simulink model "3DoFManipulatorWithBLDCM_SIMULATION"  (R2023b)
settings: Solver=VariableStepAuto  StartTime=0.0  StopTime=10  MaxStep=1e-4  RelTol=1e-3
undefined symbols (not defined in the file): X, Y, Z
libraries: spsMosfetLib x18, sm_lib x11, nesl_utility x7, eeGeneralControl x6, spsDCVoltageSourceLib x3, spsGroundLib x3, spsThreePhaseSeriesRLCBranchLib x3, spsThreePhaseVIMeasurementLib x3, slpidlib x3, sps_lib x1
(part 2 of 3)

== system 3DoFManipulatorWithBLDCM_SIMULATION/Feedforward Control/PWM LINK1 ==
  target position : Inport
  target velocity : Inport  Port=2
  actual position : Inport  Port=3
  CCW : Scope
  Duty Cycle : Scope
  MOTOR_SPEED_BLOCK3 : MATLAB Function  TreatAsAtomicUnit=on
  Mux : Mux  Inputs=2
  PID Controller Position : slpidlib/PID Controller  Controller=PID  Form=Parallel  TimeDomain=Continuous-time  UseExternalTs=off  SampleTime=-1  IntegratorMethod=Forward Euler  FilterMethod=Forward Euler  ControllerParametersSource=internal  P=800  I=20000  UseKiTs=off  D=0  N=100  UseFilter=on  TunerSelectOption=Transfer Function Based (PID Tuner App)  InitialConditionSource=internal  InitialConditionForIntegrator=0  InitialConditionForFilter=0  DifferentiatorICPrevScaledInput=0  ExternalReset=none  TrackingMode=off  Kt=1  LimitOutput=off  SatLimitsSource=internal  UpperSaturationLimit=inf  LowerSaturationLimit=-inf  LinearizeAsGain=on  AntiWindupMode=none  Kb=1  LimitIntegrator=off  UpperIntegratorSaturationLimit=inf  LowerIntegratorSaturationLimit=-inf  POutMin=[]  POutMax=[]  IOutMin=[]  IOutMax=[]  DOutMin=[]  DOutMax=[]  NOutMin=[]  NOutMax=[]  SumOutMin=[]  SumOutMax=[]  SaturationOutMin=[]  SaturationOutMax=[]  PParamMin=[]  PParamMax=[]  IParamMin=[]  IParamMax=[]  DParamMin=[]  DParamMax=[]  NParamMin=[]  NParamMax=[]  KbParamMin=[]  KbParamMax=[]  KtParamMin=[]  KtParamMax=[]  KbOutMin=[]  KbOutMax=[]  KtOutMin=[]  KtOutMax=[]  IntegratorOutMin=[]  IntegratorOutMax=[]  FilterOutMin=[]  FilterOutMax=[]  SumI1OutMin=[]  SumI1OutMax=[]  SumI2OutMin=[]  SumI2OutMax=[]  SumI3OutMin=[]  SumI3OutMax=[]  SumI4OutMin=[]  SumI4OutMax=[]  SumDOutMin=[]  SumDOutMax=[]  DifferentiatorOutMin=[]  DifferentiatorOutMax=[]  FilterDiffOutCoefMin=[]  FilterDiffOutCoefMax=[]  ReciprocalOutMin=[]  ReciprocalOutMax=[]  SumDenOutMin=[]  SumDenOutMax=[]  SumNumOutMin=[]  SumNumOutMax=[]  DivideOutMin=[]  DivideOutMax=[]  UdiffTsProdOutMin=[]  UdiffTsProdOutMax=[]  NTsProdOutMin=[]  NTsProdOutMax=[]  UintegralTsProdOutMin=[]  UintegralTsProdOutMax=[]  UngainTsProdOutMin=[]  UngainTsProdOutMax=[]  ClampingZeroOutDataTypeStr=Inherit: Inherit via back propagation  ClampingZeroOutMin=[]  ClampingZeroOutMax=[]  FilterDenConstantOutDataTypeStr=Inherit: Inherit via back propagation  FilterDenConstantOutMin=[]  FilterDenConstantOutMax=[]  PCopyOutDataTypeStr=Inherit: Inherit via back propagation  PCopyOutMin=[]  PCopyOutMax=[]  NCopyOutDataTypeStr=Inherit: Inherit via back propagation  NCopyOutMin=[]  NCopyOutMax=[]  IntegratorContinuousStateAttributes=''  IntegratorStateMustResolveToSignalObject=off  IntegratorRTWStateStorageClass=Auto  FilterContinuousStateAttributes=''  FilterStateMustResolveToSignalObject=off  FilterRTWStateStorageClass=Auto  ParallelPVariant=InternalParameters  IdealPVariant=Disabled  IVariant=InternalParameters  DVariant=InternalParameters  IntegratorVariant=Continuous  SatVariant=Disabled  AWVariant=Passthrough  PCopyVariant=Disabled  TRVariant=Disabled  FdbkBlocksVariant=Forward  IdealPFdbkVariant=Disabled  SatFdbkVariant=Disabled  DerivativeFilterVariant=ContFilter  NVariant=InternalParameters  NCopyVariant=Disabled  FilterICVariant=InternalICsFilter  IntegratorICVariant=InternalICs  ExternalResetVariant=Disabled  TRSumVariant=Passthrough  SumFdbkVariant=Disabled  SumVariant=Sum_PID  TsampFilterVariant=InternalTs  TsampNgainVariant=Passthrough  TsampIntegralVariant=Disabled_SignalSpec  ExternalSaturationOutDataTypeStr=Inherit: Same as second input
  PWM-Signal : Scope
  Variable Pulse Generator : VariablePulseGenerator  AllowZeroPulseWidth=on  SampleTime=0.1
  diff_pos : MATLAB Function  TreatAsAtomicUnit=on  SystemSampleTime=1e-4
  PWM_L1 : Outport
  wires:
  diff_pos/2(CCW) -> CCW/1, [CCW]
  diff_pos/1(diff_pos) -> PID Controller Position/1
  Mux/1 -> PWM_L1/1
  PID Controller Position/1 -> MOTOR_SPEED_BLOCK3/1(e_diff)
  Variable Pulse Generator/1 -> Mux/2, PWM-Signal/1
  MOTOR_SPEED_BLOCK3/2(p) -> Variable Pulse Generator/2
  [CCW] -> Mux/1
  MOTOR_SPEED_BLOCK3/1(dC) -> Duty Cycle/1, Variable Pulse Generator/1
  target position/1 -> diff_pos/1(t_pos)
  actual position/1 -> diff_pos/3(a_pos)
  target velocity/1 -> diff_pos/2(t_vel)

== system 3DoFManipulatorWithBLDCM_SIMULATION/Feedforward Control/PWM LINK2 ==
  target position : Inport
  target velocity : Inport  Port=2
  actual position : Inport  Port=3
  CCW : Scope
  Duty Cycle : Scope
  MOTOR_SPEED_BLOCK3 : MATLAB Function  TreatAsAtomicUnit=on
  Mux : Mux  Inputs=2
  PID Controller Position : slpidlib/PID Controller  Controller=PID  Form=Parallel  TimeDomain=Continuous-time  UseExternalTs=off  SampleTime=-1  IntegratorMethod=Forward Euler  FilterMethod=Forward Euler  ControllerParametersSource=internal  P=2000  I=20000  UseKiTs=off  D=0  N=100  UseFilter=on  TunerSelectOption=Transfer Function Based (PID Tuner App)  InitialConditionSource=internal  InitialConditionForIntegrator=0  InitialConditionForFilter=0  DifferentiatorICPrevScaledInput=0  ExternalReset=none  TrackingMode=off  Kt=1  LimitOutput=off  SatLimitsSource=internal  UpperSaturationLimit=inf  LowerSaturationLimit=-inf  LinearizeAsGain=on  AntiWindupMode=none  Kb=1  LimitIntegrator=off  UpperIntegratorSaturationLimit=inf  LowerIntegratorSaturationLimit=-inf  POutMin=[]  POutMax=[]  IOutMin=[]  IOutMax=[]  DOutMin=[]  DOutMax=[]  NOutMin=[]  NOutMax=[]  SumOutMin=[]  SumOutMax=[]  SaturationOutMin=[]  SaturationOutMax=[]  PParamMin=[]  PParamMax=[]  IParamMin=[]  IParamMax=[]  DParamMin=[]  DParamMax=[]  NParamMin=[]  NParamMax=[]  KbParamMin=[]  KbParamMax=[]  KtParamMin=[]  KtParamMax=[]  KbOutMin=[]  KbOutMax=[]  KtOutMin=[]  KtOutMax=[]  IntegratorOutMin=[]  IntegratorOutMax=[]  FilterOutMin=[]  FilterOutMax=[]  SumI1OutMin=[]  SumI1OutMax=[]  SumI2OutMin=[]  SumI2OutMax=[]  SumI3OutMin=[]  SumI3OutMax=[]  SumI4OutMin=[]  SumI4OutMax=[]  SumDOutMin=[]  SumDOutMax=[]  DifferentiatorOutMin=[]  DifferentiatorOutMax=[]  FilterDiffOutCoefMin=[]  FilterDiffOutCoefMax=[]  ReciprocalOutMin=[]  ReciprocalOutMax=[]  SumDenOutMin=[]  SumDenOutMax=[]  SumNumOutMin=[]  SumNumOutMax=[]  DivideOutMin=[]  DivideOutMax=[]  UdiffTsProdOutMin=[]  UdiffTsProdOutMax=[]  NTsProdOutMin=[]  NTsProdOutMax=[]  UintegralTsProdOutMin=[]  UintegralTsProdOutMax=[]  UngainTsProdOutMin=[]  UngainTsProdOutMax=[]  ClampingZeroOutDataTypeStr=Inherit: Inherit via back propagation  ClampingZeroOutMin=[]  ClampingZeroOutMax=[]  FilterDenConstantOutDataTypeStr=Inherit: Inherit via back propagation  FilterDenConstantOutMin=[]  FilterDenConstantOutMax=[]  PCopyOutDataTypeStr=Inherit: Inherit via back propagation  PCopyOutMin=[]  PCopyOutMax=[]  NCopyOutDataTypeStr=Inherit: Inherit via back propagation  NCopyOutMin=[]  NCopyOutMax=[]  IntegratorContinuousStateAttributes=''  IntegratorStateMustResolveToSignalObject=off  IntegratorRTWStateStorageClass=Auto  FilterContinuousStateAttributes=''  FilterStateMustResolveToSignalObject=off  FilterRTWStateStorageClass=Auto  ParallelPVariant=InternalParameters  IdealPVariant=Disabled  IVariant=InternalParameters  DVariant=InternalParameters  IntegratorVariant=Continuous  SatVariant=Disabled  AWVariant=Passthrough  PCopyVariant=Disabled  TRVariant=Disabled  FdbkBlocksVariant=Forward  IdealPFdbkVariant=Disabled  SatFdbkVariant=Disabled  DerivativeFilterVariant=ContFilter  NVariant=InternalParameters  NCopyVariant=Disabled  FilterICVariant=InternalICsFilter  IntegratorICVariant=InternalICs  ExternalResetVariant=Disabled  TRSumVariant=Passthrough  SumFdbkVariant=Disabled  SumVariant=Sum_PID  TsampFilterVariant=InternalTs  TsampNgainVariant=Passthrough  TsampIntegralVariant=Disabled_SignalSpec  ExternalSaturationOutDataTypeStr=Inherit: Same as second input
  PWM-Signal : Scope
  Variable Pulse Generator : VariablePulseGenerator  AllowZeroPulseWidth=on  SampleTime=0.1
  diff_pos : MATLAB Function  TreatAsAtomicUnit=on  SystemSampleTime=1e-4
  PWM_L2 : Outport
  wires:
  [CCW] -> Mux/1
  Variable Pulse Generator/1 -> Mux/2, PWM-Signal/1
  MOTOR_SPEED_BLOCK3/2(p) -> Variable Pulse Generator/2
  MOTOR_SPEED_BLOCK3/1(dC) -> Variable Pulse Generator/1, Duty Cycle/1
  Mux/1 -> PWM_L2/1
  PID Controller Position/1 -> MOTOR_SPEED_BLOCK3/1(e_diff)
  diff_pos/1(diff_pos) -> PID Controller Position/1
  diff_pos/2(CCW) -> CCW/1, [CCW]
  target position/1 -> diff_pos/1(t_pos)
  actual position/1 -> diff_pos/3(a_pos)
  target velocity/1 -> diff_pos/2(t_vel)

== system 3DoFManipulatorWithBLDCM_SIMULATION/Trajectorie Control/Subsystem ==
  From Workspace : FromWorkspace  VariableName=ts1_q0_pos
  From Workspace1 : FromWorkspace  VariableName=ts1_q1_pos
  From Workspace2 : FromWorkspace  VariableName=ts1_q2_pos
  From Workspace3 : FromWorkspace  VariableName=ts1_q0_vel
  From Workspace4 : FromWorkspace  VariableName=ts1_q1_vel
  From Workspace5 : FromWorkspace  VariableName=ts1_q2_vel
  From Workspace6 : FromWorkspace  VariableName=ts1_q0_acc
  From Workspace7 : FromWorkspace  VariableName=ts1_q1_acc
  From Workspace8 : FromWorkspace  VariableName=ts1_q2_acc
  Mux{,5..7} (4 alike) : Mux  Inputs=3
  Trajektorie 1 : Outport
  wires:
  From Workspace4/1 -> Mux6/2
  From Workspace3/1 -> Mux6/1
  From Workspace5/1 -> Mux6/3
  From Workspace6/1 -> Mux7/1
  From Workspace2/1 -> Mux5/3
  From Workspace8/1 -> Mux7/3
  From Workspace1/1 -> Mux5/2
  From Workspace/1 -> Mux5/1
  From Workspace7/1 -> Mux7/2
  Mux5/1 -> Mux/1
  Mux6/1 -> Mux/2
  Mux7/1 -> Mux/3
  Mux/1 -> Trajektorie 1/1

== system 3DoFManipulatorWithBLDCM_SIMULATION/Trajectorie Control/Subsystem1 ==
  From Workspace : FromWorkspace  VariableName=ts2_q0_pos
  From Workspace1 : FromWorkspace  VariableName=ts2_q1_pos
  From Workspace2 : FromWorkspace  VariableName=ts2_q2_pos
  From Workspace3 : FromWorkspace  VariableName=ts2_q0_vel
  From Workspace4 : FromWorkspace  VariableName=ts2_q1_vel
  From Workspace5 : FromWorkspace  VariableName=ts2_q2_vel
  From Workspace6 : FromWorkspace  VariableName=ts2_q0_acc
  From Workspace7 : FromWorkspace  VariableName=ts2_q1_acc
  From Workspace8 : FromWorkspace  VariableName=ts2_q2_acc
  Mux{,5..7} (4 alike) : Mux  Inputs=3
  Trajektorie 2 : Outport
  wires:
  From Workspace4/1 -> Mux6/2
  From Workspace3/1 -> Mux6/1
  From Workspace5/1 -> Mux6/3
  From Workspace6/1 -> Mux7/1
  From Workspace2/1 -> Mux5/3
  From Workspace8/1 -> Mux7/3
  From Workspace1/1 -> Mux5/2
  From Workspace/1 -> Mux5/1
  From Workspace7/1 -> Mux7/2
  Mux/1 -> Trajektorie 2/1
  Mux7/1 -> Mux/3
  Mux5/1 -> Mux/1
  Mux6/1 -> Mux/2

== system 3DoFManipulatorWithBLDCM_SIMULATION/Trajectorie Control/Subsystem2 ==
  From Workspace : FromWorkspace  VariableName=ts3_q0_pos
  From Workspace1 : FromWorkspace  VariableName=ts3_q1_pos
  From Workspace2 : FromWorkspace  VariableName=ts3_q2_pos
  From Workspace3 : FromWorkspace  VariableName=ts3_q0_vel
  From Workspace4 : FromWorkspace  VariableName=ts3_q1_vel
  From Workspace5 : FromWorkspace  VariableName=ts3_q2_vel
  From Workspace6 : FromWorkspace  VariableName=ts3_q0_acc
  From Workspace7 : FromWorkspace  VariableName=ts3_q1_acc
  From Workspace8 : FromWorkspace  VariableName=ts3_q2_acc
  Mux{,5..7} (4 alike) : Mux  Inputs=3
  Trajektorie 3 : Outport
  wires:
  From Workspace4/1 -> Mux6/2
  From Workspace3/1 -> Mux6/1
  From Workspace5/1 -> Mux6/3
  From Workspace6/1 -> Mux7/1
  From Workspace2/1 -> Mux5/3
  From Workspace8/1 -> Mux7/3
  From Workspace1/1 -> Mux5/2
  From Workspace/1 -> Mux5/1
  From Workspace7/1 -> Mux7/2
  Mux/1 -> Trajektorie 3/1
  Mux7/1 -> Mux/3
  Mux5/1 -> Mux/1
  Mux6/1 -> Mux/2

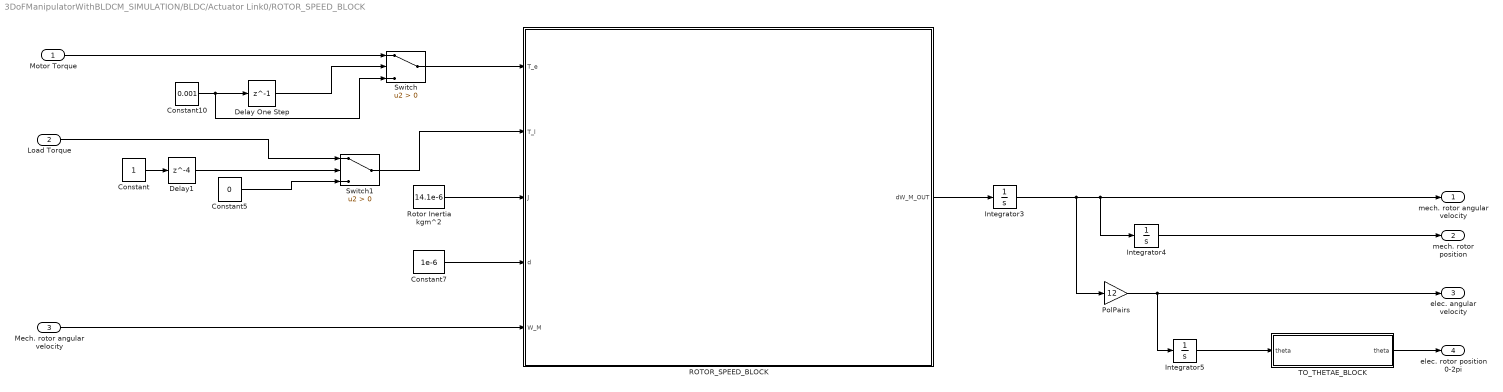
== system 3DoFManipulatorWithBLDCM_SIMULATION/BLDC/Actuator Link0/ROTOR_SPEED_BLOCK ==
  Motor Torque : Inport
  Load Torque : Inport  Port=2
  Mech. rotor angular velocity : Inport  Port=3
  Constant : Constant
  Constant10 : Constant  Value=0.001
  Constant5 : Constant  Value=0
  Constant7 : Constant  Value=1e-6
  Delay One Step : Delay  DelayLength=1
  Delay1 : Delay  DelayLength=4
  Integrator3 : Integrator
  Integrator4 : Integrator
  Integrator5 : Integrator
  PolPairs : Gain  Gain=12
  ROTOR_SPEED_BLOCK : MATLAB Function  TreatAsAtomicUnit=on
  Rotor Inertia kgm^2 : Constant  Value=14.1e-6
  Switch : Switch  Criteria=u2 > Threshold  SaturateOnIntegerOverflow=off  InputSameDT=off
  Switch1 : Switch  Criteria=u2 > Threshold  SaturateOnIntegerOverflow=off  InputSameDT=off
  TO_THETAE_BLOCK : MATLAB Function  TreatAsAtomicUnit=on
  mech. rotor angular velocity : Outport
  mech. rotor position : Outport  Port=2
  elec. angular velocity : Outport  Port=3
  elec. rotor position 0-2pi : Outport  Port=4
  wires:
  Switch1/1 -> ROTOR_SPEED_BLOCK/2(T_l)
  ROTOR_SPEED_BLOCK/1(dW_M_OUT) -> Integrator3/1
  Delay1/1 -> Switch1/2
  PolPairs/1 -> elec. angular velocity/1, Integrator5/1
  Switch/1 -> ROTOR_SPEED_BLOCK/1(T_e)
  Constant/1 -> Delay1/1
  Constant5/1 -> Switch1/3
  Delay One Step/1 -> Switch/2
  Rotor Inertia kgm^2/1 -> ROTOR_SPEED_BLOCK/3(J)
  Constant10/1 -> Delay One Step/1, Switch/3
  Integrator5/1 -> TO_THETAE_BLOCK/1("theta ")
  Constant7/1 -> ROTOR_SPEED_BLOCK/4(d)
  Motor Torque/1 -> Switch/1
  Load Torque/1 -> Switch1/1
  Integrator3/1 -> Integrator4/1, mech. rotor angular velocity/1, PolPairs/1
  Mech. rotor angular velocity/1 -> ROTOR_SPEED_BLOCK/5(W_M)
  TO_THETAE_BLOCK/1(theta) -> elec. rotor position 0-2pi/1
  Integrator4/1 -> mech. rotor position/1

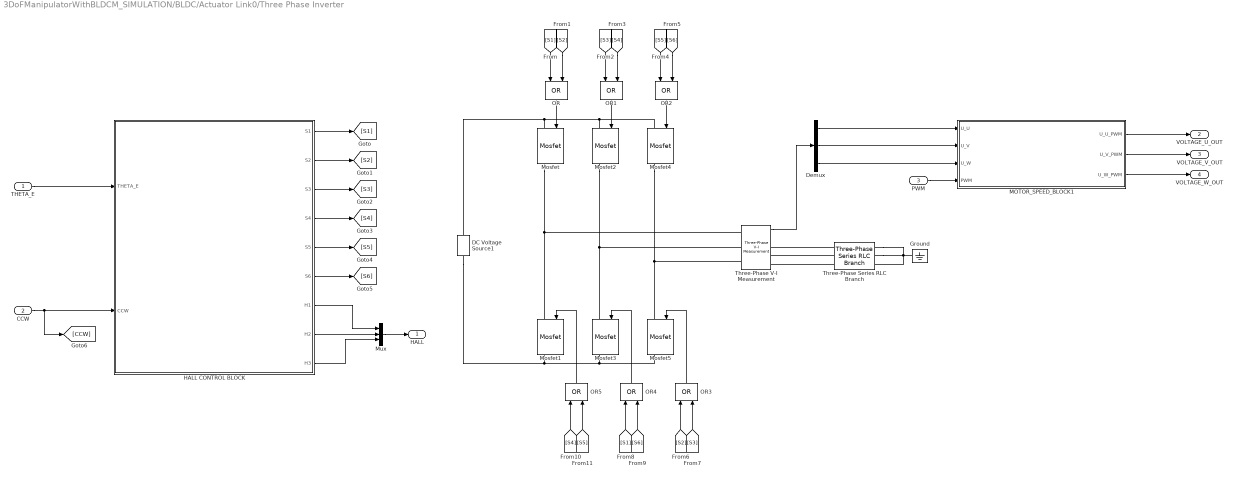
== system 3DoFManipulatorWithBLDCM_SIMULATION/BLDC/Actuator Link0/Three Phase Inverter ==
  THETA_E : Inport
  CCW : Inport  Port=2
  PWM : Inport  Port=3
  DC Voltage Source1 : spsDCVoltageSourceLib/DC Voltage Source  Amplitude=24  Measurements=None
  Demux : Demux  Outputs=3
  Ground : spsGroundLib/Ground  LConnTagsString=a
  HALL CONTROL BLOCK : MATLAB Function  TreatAsAtomicUnit=on
  MOTOR_SPEED_BLOCK1 : MATLAB Function  TreatAsAtomicUnit=on
  Mosfet{,1..5} (6 alike) : spsMosfetLib/Mosfet  Ron=0.1  Lon=0  Rd=0.01  Vfd=0  IC=0  Rs=1e5  Cs=inf  Measurements=on
  Mux : Mux  Inputs=3
  OR{,1..5} (6 alike) : Logic  Operator=OR  IconShape=distinctive  AllPortsSameDT=off  OutDataTypeStr=boolean
  Three-Phase Series RLC Branch : spsThreePhaseSeriesRLCBranchLib/Three-Phase Series RLC Branch  LConnTagsString=A|B|C  RConnTagsString=A|B|C  BranchType=RL  Resistance=100000  Inductance=0.3e-3  Capacitance=1e-6  Measurements=None
  Three-Phase V-I Measurement : spsThreePhaseVIMeasurementLib/Three-Phase V-I Measurement  VoltageMeasurement=phase-to-ground  SetLabelV=off  LabelV=Vabc  Vpu=off  VpuLL=off  CurrentMeasurement=yes  SetLabelI=off  LabelI=Iabc  Ipu=off  Pbase=100e6  Vbase=500e3  OutputType=Complex  PhasorSimulation=off  PSBequivalent=0
  HALL : Outport
  VOLTAGE_U_OUT : Outport  Port=2
  VOLTAGE_V_OUT : Outport  Port=3
  VOLTAGE_W_OUT : Outport  Port=4
  wires:
  Three-Phase V-I Measurement/1 -> Demux/1
  Demux/1 -> MOTOR_SPEED_BLOCK1/1(U_U)
  Demux/2 -> MOTOR_SPEED_BLOCK1/2(U_V)
  Demux/3 -> MOTOR_SPEED_BLOCK1/3(U_W)
  OR/1 -> Mosfet/1
  HALL CONTROL BLOCK/1(S1) -> [S1]
  [S1] -> OR/1
  HALL CONTROL BLOCK/2(S2) -> [S2]
  [S2] -> OR/2
  [S4] -> OR1/2
  [S3] -> OR1/1
  OR1/1 -> Mosfet2/1
  [S6] -> OR2/2
  [S5] -> OR2/1
  OR2/1 -> Mosfet4/1
  HALL CONTROL BLOCK/4(S4) -> [S4]
  HALL CONTROL BLOCK/3(S3) -> [S3]
  HALL CONTROL BLOCK/5(S5) -> [S5]
  HALL CONTROL BLOCK/6(S6) -> [S6]
  [S3] -> OR3/2
  [S4] -> OR5/1
  [S5] -> OR5/2
  [S6] -> OR4/2
  [S2] -> OR3/1
  [S1] -> OR4/1
  OR5/1 -> Mosfet1/1
  OR4/1 -> Mosfet3/1
  OR3/1 -> Mosfet5/1
  THETA_E/1 -> HALL CONTROL BLOCK/1(THETA_E)
  HALL CONTROL BLOCK/7(H1) -> Mux/1
  HALL CONTROL BLOCK/8(H2) -> Mux/2
  HALL CONTROL BLOCK/9(H3) -> Mux/3
  Mux/1 -> HALL/1
  MOTOR_SPEED_BLOCK1/1(U_U_PWM) -> VOLTAGE_U_OUT/1
  MOTOR_SPEED_BLOCK1/3(U_W_PWM) -> VOLTAGE_W_OUT/1
  MOTOR_SPEED_BLOCK1/2(U_V_PWM) -> VOLTAGE_V_OUT/1
  CCW/1 -> [CCW], HALL CONTROL BLOCK/2(CCW)
  PWM/1 -> MOTOR_SPEED_BLOCK1/4(PWM)
  connections:
  Three-Phase V-I Measurement/LConn3 -- Mosfet5/LConn1 -- Mosfet4/RConn1
  Mosfet1/RConn1 -- DC Voltage Source1/LConn1 -- Mosfet5/RConn1 -- Mosfet3/RConn1
  Mosfet/LConn1 -- DC Voltage Source1/RConn1 -- Mosfet4/LConn1 -- Mosfet2/LConn1
  Mosfet1/LConn1 -- Mosfet/RConn1 -- Three-Phase V-I Measurement/LConn1
  Three-Phase V-I Measurement/LConn2 -- Mosfet3/LConn1 -- Mosfet2/RConn1
  Three-Phase Series RLC Branch/RConn3 -- Three-Phase Series RLC Branch/RConn2 -- Ground/LConn1 -- Three-Phase Series RLC Branch/RConn1
  Three-Phase Series RLC Branch/LConn1 -- Three-Phase V-I Measurement/RConn1
  Three-Phase Series RLC Branch/LConn2 -- Three-Phase V-I Measurement/RConn2
  Three-Phase Series RLC Branch/LConn3 -- Three-Phase V-I Measurement/RConn3

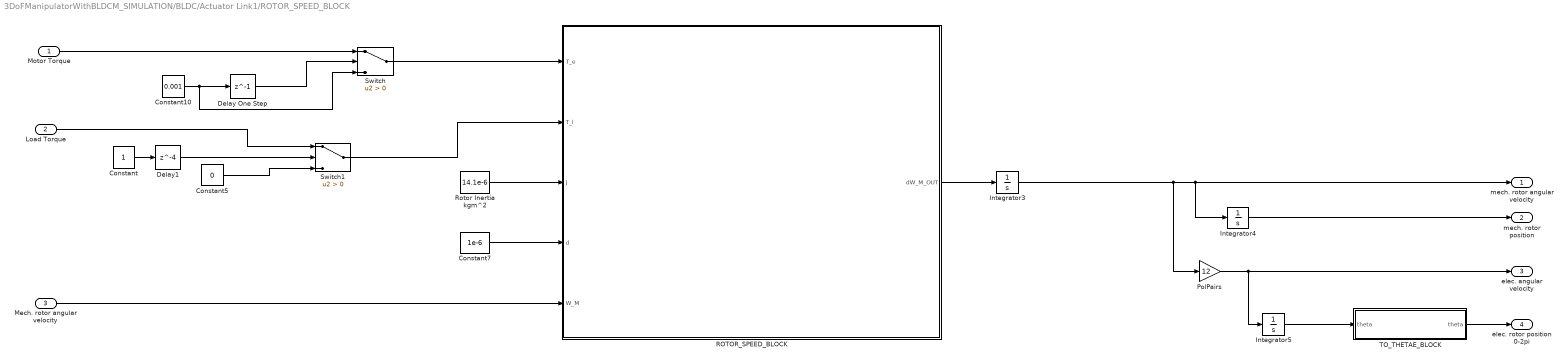
== system 3DoFManipulatorWithBLDCM_SIMULATION/BLDC/Actuator Link1/ROTOR_SPEED_BLOCK ==
  Motor Torque : Inport
  Load Torque : Inport  Port=2
  Mech. rotor angular velocity : Inport  Port=3
  Constant : Constant
  Constant10 : Constant  Value=0.001
  Constant5 : Constant  Value=0
  Constant7 : Constant  Value=1e-6
  Delay One Step : Delay  DelayLength=1
  Delay1 : Delay  DelayLength=4
  Integrator3 : Integrator
  Integrator4 : Integrator
  Integrator5 : Integrator
  PolPairs : Gain  Gain=12
  ROTOR_SPEED_BLOCK : MATLAB Function  TreatAsAtomicUnit=on
  Rotor Inertia kgm^2 : Constant  Value=14.1e-6
  Switch : Switch  Criteria=u2 > Threshold  SaturateOnIntegerOverflow=off  InputSameDT=off
  Switch1 : Switch  Criteria=u2 > Threshold  SaturateOnIntegerOverflow=off  InputSameDT=off
  TO_THETAE_BLOCK : MATLAB Function  TreatAsAtomicUnit=on
  mech. rotor angular velocity : Outport
  mech. rotor position : Outport  Port=2
  elec. angular velocity : Outport  Port=3
  elec. rotor position 0-2pi : Outport  Port=4
  wires:
  Switch1/1 -> ROTOR_SPEED_BLOCK/2(T_l)
  ROTOR_SPEED_BLOCK/1(dW_M_OUT) -> Integrator3/1
  Delay1/1 -> Switch1/2
  PolPairs/1 -> elec. angular velocity/1, Integrator5/1
  Switch/1 -> ROTOR_SPEED_BLOCK/1(T_e)
  Constant/1 -> Delay1/1
  Constant5/1 -> Switch1/3
  Delay One Step/1 -> Switch/2
  Rotor Inertia kgm^2/1 -> ROTOR_SPEED_BLOCK/3(J)
  Constant10/1 -> Delay One Step/1, Switch/3
  Integrator5/1 -> TO_THETAE_BLOCK/1("theta ")
  Constant7/1 -> ROTOR_SPEED_BLOCK/4(d)
  Motor Torque/1 -> Switch/1
  Load Torque/1 -> Switch1/1
  Integrator3/1 -> Integrator4/1, mech. rotor angular velocity/1, PolPairs/1
  Mech. rotor angular velocity/1 -> ROTOR_SPEED_BLOCK/5(W_M)
  TO_THETAE_BLOCK/1(theta) -> elec. rotor position 0-2pi/1
  Integrator4/1 -> mech. rotor position/1

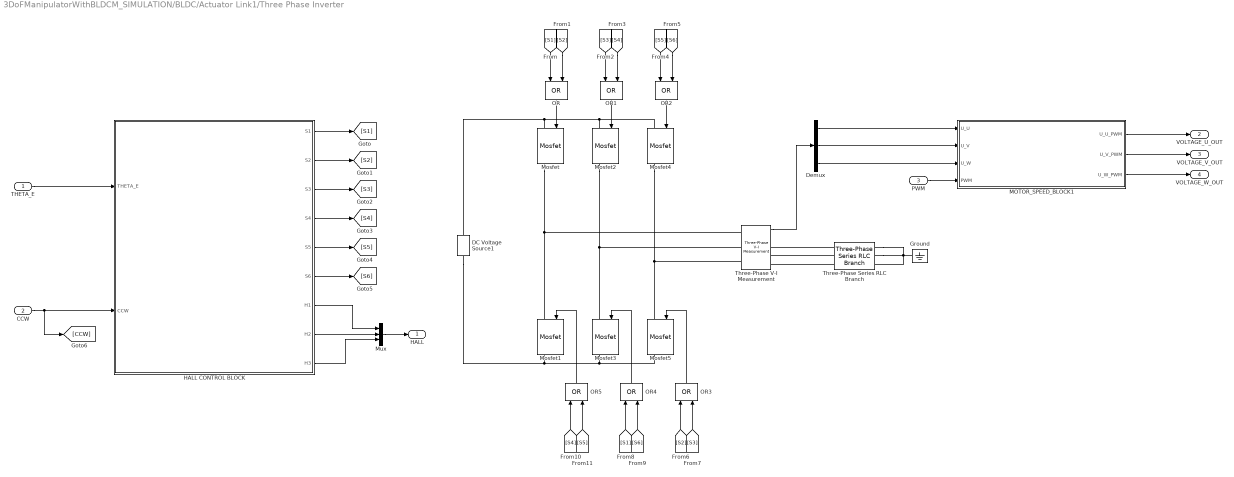
== system 3DoFManipulatorWithBLDCM_SIMULATION/BLDC/Actuator Link1/Three Phase Inverter ==
  THETA_E : Inport
  CCW : Inport  Port=2
  PWM : Inport  Port=3
  DC Voltage Source1 : spsDCVoltageSourceLib/DC Voltage Source  Amplitude=24  Measurements=None
  Demux : Demux  Outputs=3
  Ground : spsGroundLib/Ground  LConnTagsString=a
  HALL CONTROL BLOCK : MATLAB Function  TreatAsAtomicUnit=on
  MOTOR_SPEED_BLOCK1 : MATLAB Function  TreatAsAtomicUnit=on
  Mosfet{,1..5} (6 alike) : spsMosfetLib/Mosfet  Ron=0.1  Lon=0  Rd=0.01  Vfd=0  IC=0  Rs=1e5  Cs=inf  Measurements=on
  Mux : Mux  Inputs=3
  OR{,1..5} (6 alike) : Logic  Operator=OR  IconShape=distinctive  AllPortsSameDT=off  OutDataTypeStr=boolean
  Three-Phase Series RLC Branch : spsThreePhaseSeriesRLCBranchLib/Three-Phase Series RLC Branch  LConnTagsString=A|B|C  RConnTagsString=A|B|C  BranchType=RL  Resistance=100000  Inductance=0.3e-3  Capacitance=1e-6  Measurements=None
  Three-Phase V-I Measurement : spsThreePhaseVIMeasurementLib/Three-Phase V-I Measurement  VoltageMeasurement=phase-to-ground  SetLabelV=off  LabelV=Vabc  Vpu=off  VpuLL=off  CurrentMeasurement=yes  SetLabelI=off  LabelI=Iabc  Ipu=off  Pbase=100e6  Vbase=500e3  OutputType=Complex  PhasorSimulation=off  PSBequivalent=0
  HALL : Outport
  VOLTAGE_U_OUT : Outport  Port=2
  VOLTAGE_V_OUT : Outport  Port=3
  VOLTAGE_W_OUT : Outport  Port=4
  wires:
  Three-Phase V-I Measurement/1 -> Demux/1
  Demux/1 -> MOTOR_SPEED_BLOCK1/1(U_U)
  Demux/2 -> MOTOR_SPEED_BLOCK1/2(U_V)
  Demux/3 -> MOTOR_SPEED_BLOCK1/3(U_W)
  OR/1 -> Mosfet/1
  HALL CONTROL BLOCK/1(S1) -> [S1]
  [S1] -> OR/1
  HALL CONTROL BLOCK/2(S2) -> [S2]
  [S2] -> OR/2
  [S4] -> OR1/2
  [S3] -> OR1/1
  OR1/1 -> Mosfet2/1
  [S6] -> OR2/2
  [S5] -> OR2/1
  OR2/1 -> Mosfet4/1
  HALL CONTROL BLOCK/4(S4) -> [S4]
  HALL CONTROL BLOCK/3(S3) -> [S3]
  HALL CONTROL BLOCK/5(S5) -> [S5]
  HALL CONTROL BLOCK/6(S6) -> [S6]
  [S3] -> OR3/2
  [S4] -> OR5/1
  [S5] -> OR5/2
  [S6] -> OR4/2
  [S2] -> OR3/1
  [S1] -> OR4/1
  OR5/1 -> Mosfet1/1
  OR4/1 -> Mosfet3/1
  OR3/1 -> Mosfet5/1
  THETA_E/1 -> HALL CONTROL BLOCK/1(THETA_E)
  HALL CONTROL BLOCK/7(H1) -> Mux/1
  HALL CONTROL BLOCK/8(H2) -> Mux/2
  HALL CONTROL BLOCK/9(H3) -> Mux/3
  Mux/1 -> HALL/1
  MOTOR_SPEED_BLOCK1/1(U_U_PWM) -> VOLTAGE_U_OUT/1
  MOTOR_SPEED_BLOCK1/3(U_W_PWM) -> VOLTAGE_W_OUT/1
  MOTOR_SPEED_BLOCK1/2(U_V_PWM) -> VOLTAGE_V_OUT/1
  CCW/1 -> [CCW], HALL CONTROL BLOCK/2(CCW)
  PWM/1 -> MOTOR_SPEED_BLOCK1/4(PWM)
  connections:
  Three-Phase V-I Measurement/LConn3 -- Mosfet5/LConn1 -- Mosfet4/RConn1
  Mosfet1/RConn1 -- DC Voltage Source1/LConn1 -- Mosfet5/RConn1 -- Mosfet3/RConn1
  Mosfet/LConn1 -- DC Voltage Source1/RConn1 -- Mosfet4/LConn1 -- Mosfet2/LConn1
  Mosfet1/LConn1 -- Mosfet/RConn1 -- Three-Phase V-I Measurement/LConn1
  Three-Phase V-I Measurement/LConn2 -- Mosfet3/LConn1 -- Mosfet2/RConn1
  Three-Phase Series RLC Branch/RConn3 -- Three-Phase Series RLC Branch/RConn2 -- Ground/LConn1 -- Three-Phase Series RLC Branch/RConn1
  Three-Phase Series RLC Branch/LConn1 -- Three-Phase V-I Measurement/RConn1
  Three-Phase Series RLC Branch/LConn2 -- Three-Phase V-I Measurement/RConn2
  Three-Phase Series RLC Branch/LConn3 -- Three-Phase V-I Measurement/RConn3

== system 3DoFManipulatorWithBLDCM_SIMULATION/BLDC/Actuator Link2/ROTOR_SPEED_BLOCK ==
  Motor Torque : Inport
  Load Torque : Inport  Port=2
  Mech. rotor angular velocity : Inport  Port=3
  Constant : Constant
  Constant10 : Constant  Value=0.001
  Constant5 : Constant  Value=0
  Constant7 : Constant  Value=1e-6
  Delay One Step : Delay  DelayLength=1
  Delay1 : Delay  DelayLength=4
  Integrator3 : Integrator
  Integrator4 : Integrator
  Integrator5 : Integrator
  PolPairs : Gain  Gain=12
  ROTOR_SPEED_BLOCK : MATLAB Function  TreatAsAtomicUnit=on
  Rotor Inertia kgm^2 : Constant  Value=14.1e-6
  Switch : Switch  Criteria=u2 > Threshold  SaturateOnIntegerOverflow=off  InputSameDT=off
  Switch1 : Switch  Criteria=u2 > Threshold  SaturateOnIntegerOverflow=off  InputSameDT=off
  TO_THETAE_BLOCK : MATLAB Function  TreatAsAtomicUnit=on
  mech. rotor angular velocity : Outport
  mech. rotor position : Outport  Port=2
  elec. angular velocity : Outport  Port=3
  elec. rotor position 0-2pi : Outport  Port=4
  wires:
  Switch1/1 -> ROTOR_SPEED_BLOCK/2(T_l)
  ROTOR_SPEED_BLOCK/1(dW_M_OUT) -> Integrator3/1
  Delay1/1 -> Switch1/2
  PolPairs/1 -> elec. angular velocity/1, Integrator5/1
  Switch/1 -> ROTOR_SPEED_BLOCK/1(T_e)
  Constant/1 -> Delay1/1
  Constant5/1 -> Switch1/3
  Delay One Step/1 -> Switch/2
  Rotor Inertia kgm^2/1 -> ROTOR_SPEED_BLOCK/3(J)
  Constant10/1 -> Delay One Step/1, Switch/3
  Integrator5/1 -> TO_THETAE_BLOCK/1("theta ")
  Constant7/1 -> ROTOR_SPEED_BLOCK/4(d)
  Motor Torque/1 -> Switch/1
  Load Torque/1 -> Switch1/1
  Integrator3/1 -> Integrator4/1, mech. rotor angular velocity/1, PolPairs/1
  Mech. rotor angular velocity/1 -> ROTOR_SPEED_BLOCK/5(W_M)
  TO_THETAE_BLOCK/1(theta) -> elec. rotor position 0-2pi/1
  Integrator4/1 -> mech. rotor position/1

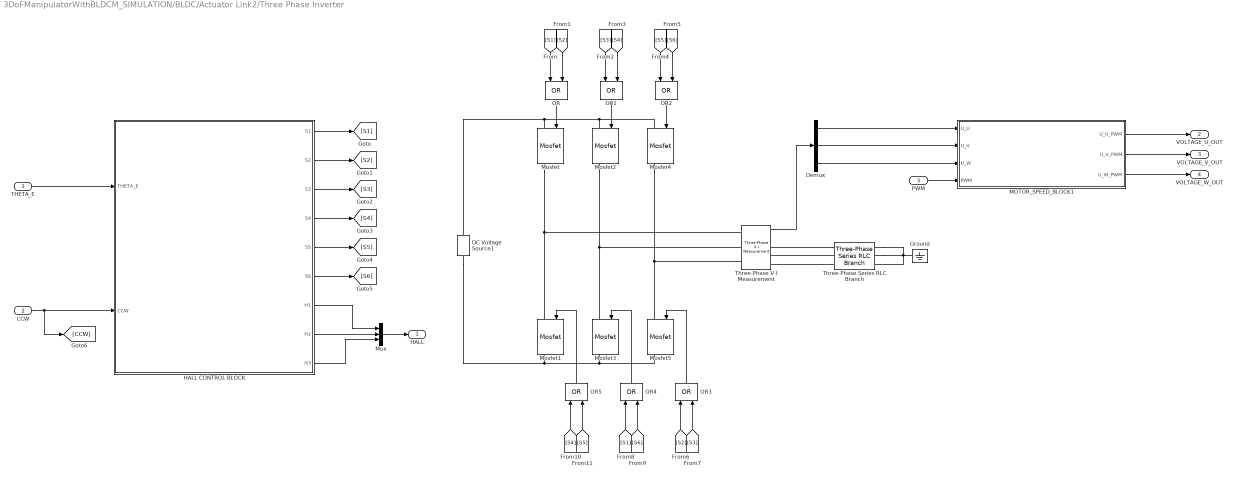
== system 3DoFManipulatorWithBLDCM_SIMULATION/BLDC/Actuator Link2/Three Phase Inverter ==
  THETA_E : Inport
  CCW : Inport  Port=2
  PWM : Inport  Port=3
  DC Voltage Source1 : spsDCVoltageSourceLib/DC Voltage Source  Amplitude=24  Measurements=None
  Demux : Demux  Outputs=3
  Ground : spsGroundLib/Ground  LConnTagsString=a
  HALL CONTROL BLOCK : MATLAB Function  TreatAsAtomicUnit=on
  MOTOR_SPEED_BLOCK1 : MATLAB Function  TreatAsAtomicUnit=on
  Mosfet{,1..5} (6 alike) : spsMosfetLib/Mosfet  Ron=0.1  Lon=0  Rd=0.01  Vfd=0  IC=0  Rs=1e5  Cs=inf  Measurements=on
  Mux : Mux  Inputs=3
  OR{,1..5} (6 alike) : Logic  Operator=OR  IconShape=distinctive  AllPortsSameDT=off  OutDataTypeStr=boolean
  Three-Phase Series RLC Branch : spsThreePhaseSeriesRLCBranchLib/Three-Phase Series RLC Branch  LConnTagsString=A|B|C  RConnTagsString=A|B|C  BranchType=RL  Resistance=100000  Inductance=0.3e-3  Capacitance=1e-6  Measurements=None
  Three-Phase V-I Measurement : spsThreePhaseVIMeasurementLib/Three-Phase V-I Measurement  VoltageMeasurement=phase-to-ground  SetLabelV=off  LabelV=Vabc  Vpu=off  VpuLL=off  CurrentMeasurement=yes  SetLabelI=off  LabelI=Iabc  Ipu=off  Pbase=100e6  Vbase=500e3  OutputType=Complex  PhasorSimulation=off  PSBequivalent=0
  HALL : Outport
  VOLTAGE_U_OUT : Outport  Port=2
  VOLTAGE_V_OUT : Outport  Port=3
  VOLTAGE_W_OUT : Outport  Port=4
  wires:
  Three-Phase V-I Measurement/1 -> Demux/1
  Demux/1 -> MOTOR_SPEED_BLOCK1/1(U_U)
  Demux/2 -> MOTOR_SPEED_BLOCK1/2(U_V)
  Demux/3 -> MOTOR_SPEED_BLOCK1/3(U_W)
  OR/1 -> Mosfet/1
  HALL CONTROL BLOCK/1(S1) -> [S1]
  [S1] -> OR/1
  HALL CONTROL BLOCK/2(S2) -> [S2]
  [S2] -> OR/2
  [S4] -> OR1/2
  [S3] -> OR1/1
  OR1/1 -> Mosfet2/1
  [S6] -> OR2/2
  [S5] -> OR2/1
  OR2/1 -> Mosfet4/1
  HALL CONTROL BLOCK/4(S4) -> [S4]
  HALL CONTROL BLOCK/3(S3) -> [S3]
  HALL CONTROL BLOCK/5(S5) -> [S5]
  HALL CONTROL BLOCK/6(S6) -> [S6]
  [S3] -> OR3/2
  [S4] -> OR5/1
  [S5] -> OR5/2
  [S6] -> OR4/2
  [S2] -> OR3/1
  [S1] -> OR4/1
  OR5/1 -> Mosfet1/1
  OR4/1 -> Mosfet3/1
  OR3/1 -> Mosfet5/1
  THETA_E/1 -> HALL CONTROL BLOCK/1(THETA_E)
  HALL CONTROL BLOCK/7(H1) -> Mux/1
  HALL CONTROL BLOCK/8(H2) -> Mux/2
  HALL CONTROL BLOCK/9(H3) -> Mux/3
  Mux/1 -> HALL/1
  MOTOR_SPEED_BLOCK1/1(U_U_PWM) -> VOLTAGE_U_OUT/1
  MOTOR_SPEED_BLOCK1/3(U_W_PWM) -> VOLTAGE_W_OUT/1
  MOTOR_SPEED_BLOCK1/2(U_V_PWM) -> VOLTAGE_V_OUT/1
  CCW/1 -> [CCW], HALL CONTROL BLOCK/2(CCW)
  PWM/1 -> MOTOR_SPEED_BLOCK1/4(PWM)
  connections:
  Three-Phase V-I Measurement/LConn3 -- Mosfet5/LConn1 -- Mosfet4/RConn1
  Mosfet1/RConn1 -- DC Voltage Source1/LConn1 -- Mosfet5/RConn1 -- Mosfet3/RConn1
  Mosfet/LConn1 -- DC Voltage Source1/RConn1 -- Mosfet4/LConn1 -- Mosfet2/LConn1
  Mosfet1/LConn1 -- Mosfet/RConn1 -- Three-Phase V-I Measurement/LConn1
  Three-Phase V-I Measurement/LConn2 -- Mosfet3/LConn1 -- Mosfet2/RConn1
  Three-Phase Series RLC Branch/RConn3 -- Three-Phase Series RLC Branch/RConn2 -- Ground/LConn1 -- Three-Phase Series RLC Branch/RConn1
  Three-Phase Series RLC Branch/LConn1 -- Three-Phase V-I Measurement/RConn1
  Three-Phase Series RLC Branch/LConn2 -- Three-Phase V-I Measurement/RConn2
  Three-Phase Series RLC Branch/LConn3 -- Three-Phase V-I Measurement/RConn3

== matlab function 3DoFManipulatorWithBLDCM_SIMULATION/BLDC/Actuator Link0/ROTOR_SPEED_BLOCK/ROTOR_SPEED_BLOCK ==
  data: T_e input; T_l input; J input; d input; dW_M_OUT output; W_M input
function dW_M_OUT = MOTOR_SPEED_BLOCK(T_e,T_l,J,d,W_M)
%#codegen

%    This function was generated by the Symbolic Math Toolbox version 23.2.
%    20-Mar-2024 19:58:52

dW_M_OUT = -(-T_e+T_l+W_M.*d)./J;
end

== matlab function 3DoFManipulatorWithBLDCM_SIMULATION/Encoder/ENCODER_BLOCK_L1 ==
  data: encoder_output output; actual_position input
function encoder_output = simulateEncoder(actual_position)

    % https://www.siko-global.com/de-de/produkte/rotoline-drehgeber/absolute-drehgeber/wh5850
    % Auflösung wäre theoretisch 200pi/2^19
    resolution = 0.0012;
    delay = 0.0001;
    dt = 2e-4;

    % quantizes
    quantized_position = round(actual_position / resolution) * resolution;

    % delay
    persistent position_queue;
    if isempty(position_queue)
        position_queue = repmat(quantized_position, 1, round(delay/dt));
    end
    encoder_output = position_queue(1)/100;
    position_queue = [position_queue(2:end), quantized_position];
    
end

== matlab function 3DoFManipulatorWithBLDCM_SIMULATION/BLDC/Actuator Link1/BACK_EMF_BLOCK ==
  data: W_M input; K_E input; THETA_E input; BEMF_U output; BEMF_V output; BEMF_W output
function [BEMF_U, BEMF_V, BEMF_W] = BEMF_BLOCK(W_M, K_E, THETA_E)
%#codegen

%    This function was generated by the Symbolic Math Toolbox version 23.2.
%    20-Mar-2024 19:08:31

%THETA = mod(THETA_E,  2*pi);
THETA = THETA_E;
% electrical theta 0°-60°
if (0 <= THETA) && (THETA < 1*pi/3)
    F_U = 1;
    F_V = -1;
    F_W = 1-6*THETA/pi;

% electrical theta 60°-120°
elseif (1*pi/3 <= THETA) &&(THETA < 2*pi/3)
    F_U = 1;
    F_V = 6*THETA/pi - 3;
    F_W = -1;

% electrical theta 120°-180°
elseif (2*pi/3 <= THETA) && (THETA < pi)
    F_U = -6*THETA/pi + 5;
    F_V = 1;
    F_W = -1;

% electrical theta 180°-240°
elseif (pi <= THETA) && (THETA < 4*pi/3)
    F_U = -1;
    F_V = 1;
    F_W = 6*THETA/pi -7;

% electrical theta 240°-300°
elseif (4*pi/3 <= THETA) && (THETA < 5*pi/3)
    F_U = -1;
    F_V = -6*THETA/pi + 9;
    F_W = 1;

% electrical theta 300°-360°
elseif (5*pi/3 <= THETA) && (THETA < 2*pi)
    F_U = 6*THETA/pi - 11;
    F_V = -1;
    F_W = 1;

% something went wrong
else
    F_U = NaN;
    F_V = NaN;
    F_W = NaN;
end

BEMF_U = K_E*W_M*F_U;
BEMF_V = K_E*W_M*F_V;
BEMF_W = K_E*W_M*F_W;

end

== matlab function 3DoFManipulatorWithBLDCM_SIMULATION/BLDC/Actuator Link0/ELECTROMAGNETIC_TORQUE_BLOCK ==
  data: I_U input; I_V input; I_W input; BEMF_U input; BEMF_V input; BEMF_W input; W_M input; T_E_OUT output; K_T input; THETA_E input; T_E_TEST output
function [T_E_OUT,T_E_TEST] = ELECTROMAGNETIC_TORQUE_BLOCK(I_U, I_V, I_W, BEMF_U, BEMF_V, BEMF_W, W_M, K_T, THETA_E)
%#codegen

%    This function was generated by the Symbolic Math Toolbox version 23.2.
%    20-Mar-2024 15:56:32

T_E_OUT = ((BEMF_U*I_U+BEMF_V*I_V+BEMF_W*I_W)./W_M);

%THETA = mod(THETA_E,  2*pi);
THETA = THETA_E;
% electrical theta 0°-60°
if (0 <= THETA) && (THETA < 1*pi/3)
    F_U = 1;
    F_V = -1;
    F_W = 1-6*THETA/pi;

% electrical theta 60°-120°
elseif (1*pi/3 <= THETA) &&(THETA < 2*pi/3)
    F_U = 1;
    F_V = 6*THETA/pi - 3;
    F_W = -1;

% electrical theta 120°-180°
elseif (2*pi/3 <= THETA) && (THETA < pi)
    F_U = -6*THETA/pi + 5;
    F_V = 1;
    F_W = -1;

% electrical theta 180°-240°
elseif (pi <= THETA) && (THETA < 4*pi/3)
    F_U = -1;
    F_V = 1;
    F_W = 6*THETA/pi -7;

% electrical theta 240°-300°
elseif (4*pi/3 <= THETA) && (THETA < 5*pi/3)
    F_U = -1;
    F_V = -6*THETA/pi + 9;
    F_W = 1;

% electrical theta 300°-360°
elseif (5*pi/3 <= THETA) && (THETA < 2*pi)
    F_U = 6*THETA/pi - 11;
    F_V = -1;
    F_W = 1;

% something went wrong
else
    F_U = NaN;
    F_V = NaN;
    F_W = NaN;
end

T_E_TEST = K_T*((F_U*I_U)+(F_V*I_V)+(F_W*I_W));

end

== matlab function 3DoFManipulatorWithBLDCM_SIMULATION/BLDC/Actuator Link1/CURRENT_BLOCK ==
  data: I_U input; dI_U_OUT output; I_V input; U_U input; U_V input; U_W input; L input; R input; BEMF_U input; BEMF_V input; BEMF_W input; dI_V_OUT output; dI_W_OUT output
function [dI_U_OUT,dI_V_OUT,dI_W_OUT] = CURRENT_BLOCK(I_U,I_V,U_U,U_V,U_W,L,R,BEMF_U,BEMF_V,BEMF_W)
%#codegen

%    This function was generated by the Symbolic Math Toolbox version 23.2.
%    20-Mar-2024 19:08:31

% https://de.mathworks.com/matlabcentral/answers/446003-relation-between-flux-linkage-and-voltage-constant-power_pmsynchronousmachineparams
% based on the link the magnetic flux is approximately lamda
%LAMDA = (sqrt(2)/sqrt(3)) * ((48/sqrt(2))/P*W_M)
%LAMDA = 1/sqrt(3) * (K_T/1000*P) * (60/2*pi)

%U_UV = U_U - U_V;
%U_VW = U_V - U_W;

%dI_U_OUT = (U_UV.*2.0+U_VW-I_U.*R.*3.0+P*MFLUX*W_M*(-EMF_U.*2.0+EMF_V+EMF_W))./(L.*3.0);

%dI_V_OUT = (-U_UV+U_VW-I_V.*R.*3.0+P*MFLUX*W_M*(EMF_U-EMF_V.*2.0+EMF_W))./(L.*3.0);

%dI_W_OUT = -(dI_U_OUT+dI_V_OUT);

E_UW = BEMF_U - BEMF_W;
E_WV = BEMF_W - BEMF_V;

U_UW = U_U - U_W;
U_WV = U_W - U_V;

dI_U_OUT = (U_UW.*2.0 + U_WV - I_U.*R.*3.0 - E_UW.*2.0 - E_WV)./(L.*3.0);
dI_V_OUT = (-U_UW - U_WV.*2.0 - I_V.*R.*3.0 + E_UW + E_WV.*2.0)./(L.*3.0);
dI_W_OUT = -(dI_U_OUT+dI_V_OUT);

%dI_U_OUT = -(R*I_U)/L - (P*W_M*EMF_U)/(2*L) + U_U/L
%dI_V_OUT = -(R*I_V)/L - (P*W_M*EMF_V)/(2*L) + U_V/L
%dI_W_OUT = -(R*I_W)/L - (P*W_M*EMF_W)/(2*L) + U_W/L
%dI_W_OUT = -(dI_U_OUT+dI_V_OUT)
end

== matlab function 3DoFManipulatorWithBLDCM_SIMULATION/BLDC/Actuator Link1/ELECTROMAGNETIC_TORQUE_BLOCK ==
  data: I_U input; I_V input; I_W input; BEMF_U input; BEMF_V input; BEMF_W input; W_M input; T_E_OUT output; K_T input; THETA_E input; T_E_TEST output
function [T_E_OUT,T_E_TEST] = ELECTROMAGNETIC_TORQUE_BLOCK(I_U, I_V, I_W, BEMF_U, BEMF_V, BEMF_W, W_M, K_T, THETA_E)
%#codegen

%    This function was generated by the Symbolic Math Toolbox version 23.2.
%    20-Mar-2024 15:56:32

T_E_OUT = ((BEMF_U*I_U+BEMF_V*I_V+BEMF_W*I_W)./W_M);

%THETA = mod(THETA_E,  2*pi);
THETA = THETA_E;
% electrical theta 0°-60°
if (0 <= THETA) && (THETA < 1*pi/3)
    F_U = 1;
    F_V = -1;
    F_W = 1-6*THETA/pi;

% electrical theta 60°-120°
elseif (1*pi/3 <= THETA) &&(THETA < 2*pi/3)
    F_U = 1;
    F_V = 6*THETA/pi - 3;
    F_W = -1;

% electrical theta 120°-180°
elseif (2*pi/3 <= THETA) && (THETA < pi)
    F_U = -6*THETA/pi + 5;
    F_V = 1;
    F_W = -1;

% electrical theta 180°-240°
elseif (pi <= THETA) && (THETA < 4*pi/3)
    F_U = -1;
    F_V = 1;
    F_W = 6*THETA/pi -7;

% electrical theta 240°-300°
elseif (4*pi/3 <= THETA) && (THETA < 5*pi/3)
    F_U = -1;
    F_V = -6*THETA/pi + 9;
    F_W = 1;

% electrical theta 300°-360°
elseif (5*pi/3 <= THETA) && (THETA < 2*pi)
    F_U = 6*THETA/pi - 11;
    F_V = -1;
    F_W = 1;

% something went wrong
else
    F_U = NaN;
    F_V = NaN;
    F_W = NaN;
end

T_E_TEST = K_T*((F_U*I_U)+(F_V*I_V)+(F_W*I_W));

end

== matlab function 3DoFManipulatorWithBLDCM_SIMULATION/BLDC/Actuator Link1/ROTOR_SPEED_BLOCK/ROTOR_SPEED_BLOCK ==
  data: T_e input; T_l input; J input; d input; dW_M_OUT output; W_M input
function dW_M_OUT = MOTOR_SPEED_BLOCK(T_e,T_l,J,d,W_M)
%#codegen

%    This function was generated by the Symbolic Math Toolbox version 23.2.
%    20-Mar-2024 19:58:52

dW_M_OUT = -(-T_e+T_l+W_M.*d)./J;
end

== matlab function 3DoFManipulatorWithBLDCM_SIMULATION/BLDC/Actuator Link1/ROTOR_SPEED_BLOCK/TO_THETAE_BLOCK ==
  data: theta output; theta input
function theta = generateTheta(theta)
    theta = mod(theta, 2*pi);
end

== matlab function 3DoFManipulatorWithBLDCM_SIMULATION/Encoder/ENCODER_BLOCK_L2 ==
  data: encoder_output output; actual_position input
function encoder_output = simulateEncoder(actual_position)

    % https://www.siko-global.com/de-de/produkte/rotoline-drehgeber/absolute-drehgeber/wh5850
    % Auflösung wäre theoretisch 200pi/2^19
    resolution = 0.0012;
    delay = 0.0001;
    dt = 2e-4;

    % quantizes
    quantized_position = round(actual_position / resolution) * resolution;

    % delay
    persistent position_queue;
    if isempty(position_queue)
        position_queue = repmat(quantized_position, 1, round(delay/dt));
    end
    encoder_output = position_queue(1)/100;
    position_queue = [position_queue(2:end), quantized_position];
    
end

== matlab function 3DoFManipulatorWithBLDCM_SIMULATION/BLDC/Actuator Link2/BACK_EMF_BLOCK ==
  data: W_M input; K_E input; THETA_E input; BEMF_U output; BEMF_V output; BEMF_W output
function [BEMF_U, BEMF_V, BEMF_W] = BEMF_BLOCK(W_M, K_E, THETA_E)
%#codegen

%    This function was generated by the Symbolic Math Toolbox version 23.2.
%    20-Mar-2024 19:08:31

%THETA = mod(THETA_E,  2*pi);
THETA = THETA_E;
% electrical theta 0°-60°
if (0 <= THETA) && (THETA < 1*pi/3)
    F_U = 1;
    F_V = -1;
    F_W = 1-6*THETA/pi;

% electrical theta 60°-120°
elseif (1*pi/3 <= THETA) &&(THETA < 2*pi/3)
    F_U = 1;
    F_V = 6*THETA/pi - 3;
    F_W = -1;

% electrical theta 120°-180°
elseif (2*pi/3 <= THETA) && (THETA < pi)
    F_U = -6*THETA/pi + 5;
    F_V = 1;
    F_W = -1;

% electrical theta 180°-240°
elseif (pi <= THETA) && (THETA < 4*pi/3)
    F_U = -1;
    F_V = 1;
    F_W = 6*THETA/pi -7;

% electrical theta 240°-300°
elseif (4*pi/3 <= THETA) && (THETA < 5*pi/3)
    F_U = -1;
    F_V = -6*THETA/pi + 9;
    F_W = 1;

% electrical theta 300°-360°
elseif (5*pi/3 <= THETA) && (THETA < 2*pi)
    F_U = 6*THETA/pi - 11;
    F_V = -1;
    F_W = 1;

% something went wrong
else
    F_U = NaN;
    F_V = NaN;
    F_W = NaN;
end

BEMF_U = K_E*W_M*F_U;
BEMF_V = K_E*W_M*F_V;
BEMF_W = K_E*W_M*F_W;

end

== matlab function 3DoFManipulatorWithBLDCM_SIMULATION/BLDC/Actuator Link2/CURRENT_BLOCK ==
  data: I_U input; dI_U_OUT output; I_V input; U_U input; U_V input; U_W input; L input; R input; BEMF_U input; BEMF_V input; BEMF_W input; dI_V_OUT output; dI_W_OUT output
function [dI_U_OUT,dI_V_OUT,dI_W_OUT] = CURRENT_BLOCK(I_U,I_V,U_U,U_V,U_W,L,R,BEMF_U,BEMF_V,BEMF_W)
%#codegen

%    This function was generated by the Symbolic Math Toolbox version 23.2.
%    20-Mar-2024 19:08:31

% https://de.mathworks.com/matlabcentral/answers/446003-relation-between-flux-linkage-and-voltage-constant-power_pmsynchronousmachineparams
% based on the link the magnetic flux is approximately lamda
%LAMDA = (sqrt(2)/sqrt(3)) * ((48/sqrt(2))/P*W_M)
%LAMDA = 1/sqrt(3) * (K_T/1000*P) * (60/2*pi)

%U_UV = U_U - U_V;
%U_VW = U_V - U_W;

%dI_U_OUT = (U_UV.*2.0+U_VW-I_U.*R.*3.0+P*MFLUX*W_M*(-EMF_U.*2.0+EMF_V+EMF_W))./(L.*3.0);

%dI_V_OUT = (-U_UV+U_VW-I_V.*R.*3.0+P*MFLUX*W_M*(EMF_U-EMF_V.*2.0+EMF_W))./(L.*3.0);

%dI_W_OUT = -(dI_U_OUT+dI_V_OUT);

E_UW = BEMF_U - BEMF_W;
E_WV = BEMF_W - BEMF_V;

U_UW = U_U - U_W;
U_WV = U_W - U_V;

dI_U_OUT = (U_UW.*2.0 + U_WV - I_U.*R.*3.0 - E_UW.*2.0 - E_WV)./(L.*3.0);
dI_V_OUT = (-U_UW - U_WV.*2.0 - I_V.*R.*3.0 + E_UW + E_WV.*2.0)./(L.*3.0);
dI_W_OUT = -(dI_U_OUT+dI_V_OUT);

%dI_U_OUT = -(R*I_U)/L - (P*W_M*EMF_U)/(2*L) + U_U/L
%dI_V_OUT = -(R*I_V)/L - (P*W_M*EMF_V)/(2*L) + U_V/L
%dI_W_OUT = -(R*I_W)/L - (P*W_M*EMF_W)/(2*L) + U_W/L
%dI_W_OUT = -(dI_U_OUT+dI_V_OUT)
end

== matlab function 3DoFManipulatorWithBLDCM_SIMULATION/BLDC/Actuator Link2/ELECTROMAGNETIC_TORQUE_BLOCK ==
  data: I_U input; I_V input; I_W input; BEMF_U input; BEMF_V input; BEMF_W input; W_M input; T_E_OUT output; K_T input; THETA_E input; T_E_TEST output
function [T_E_OUT,T_E_TEST] = ELECTROMAGNETIC_TORQUE_BLOCK(I_U, I_V, I_W, BEMF_U, BEMF_V, BEMF_W, W_M, K_T, THETA_E)
%#codegen

%    This function was generated by the Symbolic Math Toolbox version 23.2.
%    20-Mar-2024 15:56:32

T_E_OUT = ((BEMF_U*I_U+BEMF_V*I_V+BEMF_W*I_W)./W_M);

%THETA = mod(THETA_E,  2*pi);
THETA = THETA_E;
% electrical theta 0°-60°
if (0 <= THETA) && (THETA < 1*pi/3)
    F_U = 1;
    F_V = -1;
    F_W = 1-6*THETA/pi;

% electrical theta 60°-120°
elseif (1*pi/3 <= THETA) &&(THETA < 2*pi/3)
    F_U = 1;
    F_V = 6*THETA/pi - 3;
    F_W = -1;

% electrical theta 120°-180°
elseif (2*pi/3 <= THETA) && (THETA < pi)
    F_U = -6*THETA/pi + 5;
    F_V = 1;
    F_W = -1;

% electrical theta 180°-240°
elseif (pi <= THETA) && (THETA < 4*pi/3)
    F_U = -1;
    F_V = 1;
    F_W = 6*THETA/pi -7;

% electrical theta 240°-300°
elseif (4*pi/3 <= THETA) && (THETA < 5*pi/3)
    F_U = -1;
    F_V = -6*THETA/pi + 9;
    F_W = 1;

% electrical theta 300°-360°
elseif (5*pi/3 <= THETA) && (THETA < 2*pi)
    F_U = 6*THETA/pi - 11;
    F_V = -1;
    F_W = 1;

% something went wrong
else
    F_U = NaN;
    F_V = NaN;
    F_W = NaN;
end

T_E_TEST = K_T*((F_U*I_U)+(F_V*I_V)+(F_W*I_W));

end

== matlab function 3DoFManipulatorWithBLDCM_SIMULATION/BLDC/Actuator Link2/ROTOR_SPEED_BLOCK/ROTOR_SPEED_BLOCK ==
  data: T_e input; T_l input; J input; d input; dW_M_OUT output; W_M input
function dW_M_OUT = MOTOR_SPEED_BLOCK(T_e,T_l,J,d,W_M)
%#codegen

%    This function was generated by the Symbolic Math Toolbox version 23.2.
%    20-Mar-2024 19:58:52

dW_M_OUT = -(-T_e+T_l+W_M.*d)./J;
end

== matlab function 3DoFManipulatorWithBLDCM_SIMULATION/BLDC/Actuator Link2/ROTOR_SPEED_BLOCK/TO_THETAE_BLOCK ==
  data: theta output; theta input
function theta = generateTheta(theta)
    theta = mod(theta, 2*pi);
end

== matlab function 3DoFManipulatorWithBLDCM_SIMULATION/BLDC/Actuator Link1/Three Phase Inverter/HALL CONTROL BLOCK ==
  data: S1 output; S2 output; S3 output; S4 output; S5 output; S6 output; THETA_E input; H1 output; H2 output; H3 output; CCW input
function [S1, S2, S3, S4, S5, S6, H1, H2 ,H3] = HALL_BLOCK(THETA_E, CCW)
%#codegen

% Normalisierung
%THETA_E = mod(THETA_E, 2*pi);
% Initialisieren Sie alle Signale auf 0

THETA = mod(THETA_E,  2*pi);

% electrical theta 0°-60°
if (0 <= THETA) && (THETA < 1*pi/3)
    H1 = 1;
    H2 = 0;
    H3 = 1;

% electrical theta 60°-120°
elseif (1*pi/3 <= THETA) &&(THETA < 2*pi/3)
    H1 = 1;
    H2 = 0;
    H3 = 0;
% electrical theta 120°-180°
elseif (2*pi/3 <= THETA) && (THETA < pi)
    H1 = 1;
    H2 = 1;
    H3 = 0;

% electrical theta 180°-240°
elseif (pi <= THETA) && (THETA < 4*pi/3)
    H1 = 0;
    H2 = 1;
    H3 = 0;

% electrical theta 240°-300°
elseif (4*pi/3 <= THETA) && (THETA < 5*pi/3)
    H1 = 0;
    H2 = 1;
    H3 = 1;

% electrical theta 300°-360°
elseif (5*pi/3 <= THETA) && (THETA < 2*pi)
    H1 = 0;
    H2 = 0;
    H3 = 1;

% something went wrong
else
    H1 = 0;
    H2 = 0;
    H3 = 0;
end

if CCW ~= 1
    if (H1 == 1) && (H3 == 1)
       S3 = 0; S2 = 0; S4 = 0; S5 = 0; S6 = 0;
       S1 = 1;
    elseif (H1 == 1) && (H2 ~= 1 && H3 ~= 1)
       S1 = 0; S4 = 0; S3 = 0; S5 = 0; S6 = 0;
       S2 = 1;
    elseif (H1 == 1) && (H2 == 1)
       S1 = 0; S2 = 0; S5 = 0; S4 = 0; S6 = 0;
       S3 = 1;
    elseif (H2 == 1) && (H1 ~= 1 && H3 ~= 1)
       S1 = 0; S2 = 0; S3 = 0; S6 = 0; S5 = 0;
       S4 = 1;
    elseif (H2 == 1) && (H3 == 1)
       S2 = 0; S3 = 0; S4 = 0; S1 = 0; S6 = 0;
       S5 = 1;
    elseif (H3 == 1) && (H1 ~= 1 && H2 ~= 1)
       S1 = 0; S3 = 0; S4 = 0; S5 = 0; S2 = 0;
       S6 = 1;
    else
       S1 = 0; S2 = 0; S3 = 0; S4 = 0; S5 = 0; S6 = 0; 
    end
else
    if (H1 == 1) && (H3 == 1)
       S3 = 0; S2 = 0; S1 = 0; S5 = 0; S6 = 0;
       S4 = 1;
    elseif (H1 == 1) && (H2 ~= 1 && H3 ~= 1)
       S1 = 0; S4 = 0; S3 = 0; S2 = 0; S6 = 0;
       S5 = 1;
    elseif (H1 == 1) && (H2 == 1)
       S1 = 0; S2 = 0; S5 = 0; S4 = 0; S3 = 0;
       S6 = 1;
    elseif (H2 == 1) && (H1 ~= 1 && H3 ~= 1)
       S4 = 0; S2 = 0; S3 = 0; S6 = 0; S5 = 0;
       S1 = 1;
    elseif (H2 == 1) && (H3 == 1)
       S5 = 0; S3 = 0; S4 = 0; S1 = 0; S6 = 0;
       S2 = 1;
    elseif (H3 == 1) && (H1 ~= 1 && H2 ~= 1)
       S1 = 0; S6 = 0; S4 = 0; S5 = 0; S2 = 0;
       S3 = 1;
    else
       S1 = 0; S2 = 0; S3 = 0; S4 = 0; S5 = 0; S6 = 0; 
    end
end

end

== matlab function 3DoFManipulatorWithBLDCM_SIMULATION/BLDC/TO_THETAE_BLOCK ==
  data: theta output; theta input
function theta = generateTheta(theta)
    theta = mod(theta, 2*pi);
end

== matlab function 3DoFManipulatorWithBLDCM_SIMULATION/Tracking Position Error/forward Kinematic ==
  data: q0a input; q1a input; q2a input; actualCartesianPosition output; q0t input; q1t input; q2t input; targetCartesianPosition output
function [actualCartesianPosition, targetCartesianPosition] = forwardKinematics(q0a, q1a, q2a, q0t, q1t, q2t)

l0 = 500;
l1 = 1000;
l2 = 1000;

actualCartesianPosition = [cos(q0a)*(l1*cos(q1a)+l2*cos(q1a+q2a));
                            sin(q0a)*(l1*cos(q1a)+l2*cos(q1a+q2a));
                            l0+l1*sin(q1a)+l2*sin(q1a+q2a)];

targetCartesianPosition = [cos(q0t)*(l1*cos(q1t)+l2*cos(q1t+q2t));
                            sin(q0t)*(l1*cos(q1t)+l2*cos(q1t+q2t));
                            l0+l1*sin(q1t)+l2*sin(q1t+q2t)];

end

== matlab function 3DoFManipulatorWithBLDCM_SIMULATION/BLDC/Actuator Link0/Three Phase Inverter/HALL CONTROL BLOCK ==
  data: S1 output; S2 output; S3 output; S4 output; S5 output; S6 output; THETA_E input; H1 output; H2 output; H3 output; CCW input
function [S1, S2, S3, S4, S5, S6, H1, H2 ,H3] = HALL_BLOCK(THETA_E, CCW)
%#codegen

% Normalisierung
%THETA_E = mod(THETA_E, 2*pi);
% Initialisieren Sie alle Signale auf 0

THETA = mod(THETA_E,  2*pi);

% electrical theta 0°-60°
if (0 <= THETA) && (THETA < 1*pi/3)
    H1 = 1;
    H2 = 0;
    H3 = 1;

% electrical theta 60°-120°
elseif (1*pi/3 <= THETA) &&(THETA < 2*pi/3)
    H1 = 1;
    H2 = 0;
    H3 = 0;
% electrical theta 120°-180°
elseif (2*pi/3 <= THETA) && (THETA < pi)
    H1 = 1;
    H2 = 1;
    H3 = 0;

% electrical theta 180°-240°
elseif (pi <= THETA) && (THETA < 4*pi/3)
    H1 = 0;
    H2 = 1;
    H3 = 0;

% electrical theta 240°-300°
elseif (4*pi/3 <= THETA) && (THETA < 5*pi/3)
    H1 = 0;
    H2 = 1;
    H3 = 1;

% electrical theta 300°-360°
elseif (5*pi/3 <= THETA) && (THETA < 2*pi)
    H1 = 0;
    H2 = 0;
    H3 = 1;

% something went wrong
else
    H1 = 0;
    H2 = 0;
    H3 = 0;
end

if CCW ~= 1
    if (H1 == 1) && (H3 == 1)
       S3 = 0; S2 = 0; S4 = 0; S5 = 0; S6 = 0;
       S1 = 1;
    elseif (H1 == 1) && (H2 ~= 1 && H3 ~= 1)
       S1 = 0; S4 = 0; S3 = 0; S5 = 0; S6 = 0;
       S2 = 1;
    elseif (H1 == 1) && (H2 == 1)
       S1 = 0; S2 = 0; S5 = 0; S4 = 0; S6 = 0;
       S3 = 1;
    elseif (H2 == 1) && (H1 ~= 1 && H3 ~= 1)
       S1 = 0; S2 = 0; S3 = 0; S6 = 0; S5 = 0;
       S4 = 1;
    elseif (H2 == 1) && (H3 == 1)
       S2 = 0; S3 = 0; S4 = 0; S1 = 0; S6 = 0;
       S5 = 1;
    elseif (H3 == 1) && (H1 ~= 1 && H2 ~= 1)
       S1 = 0; S3 = 0; S4 = 0; S5 = 0; S2 = 0;
       S6 = 1;
    else
       S1 = 0; S2 = 0; S3 = 0; S4 = 0; S5 = 0; S6 = 0; 
    end
else
    if (H1 == 1) && (H3 == 1)
       S3 = 0; S2 = 0; S1 = 0; S5 = 0; S6 = 0;
       S4 = 1;
    elseif (H1 == 1) && (H2 ~= 1 && H3 ~= 1)
       S1 = 0; S4 = 0; S3 = 0; S2 = 0; S6 = 0;
       S5 = 1;
    elseif (H1 == 1) && (H2 == 1)
       S1 = 0; S2 = 0; S5 = 0; S4 = 0; S3 = 0;
       S6 = 1;
    elseif (H2 == 1) && (H1 ~= 1 && H3 ~= 1)
       S4 = 0; S2 = 0; S3 = 0; S6 = 0; S5 = 0;
       S1 = 1;
    elseif (H2 == 1) && (H3 == 1)
       S5 = 0; S3 = 0; S4 = 0; S1 = 0; S6 = 0;
       S2 = 1;
    elseif (H3 == 1) && (H1 ~= 1 && H2 ~= 1)
       S1 = 0; S6 = 0; S4 = 0; S5 = 0; S2 = 0;
       S3 = 1;
    else
       S1 = 0; S2 = 0; S3 = 0; S4 = 0; S5 = 0; S6 = 0; 
    end
end

end

== matlab function 3DoFManipulatorWithBLDCM_SIMULATION/BLDC/Actuator Link2/Three Phase Inverter/HALL CONTROL BLOCK ==
  data: S1 output; S2 output; S3 output; S4 output; S5 output; S6 output; THETA_E input; H1 output; H2 output; H3 output; CCW input
function [S1, S2, S3, S4, S5, S6, H1, H2 ,H3] = HALL_BLOCK(THETA_E, CCW)
%#codegen

% Normalisierung
%THETA_E = mod(THETA_E, 2*pi);
% Initialisieren Sie alle Signale auf 0

THETA = mod(THETA_E,  2*pi);

% electrical theta 0°-60°
if (0 <= THETA) && (THETA < 1*pi/3)
    H1 = 1;
    H2 = 0;
    H3 = 1;

% electrical theta 60°-120°
elseif (1*pi/3 <= THETA) &&(THETA < 2*pi/3)
    H1 = 1;
    H2 = 0;
    H3 = 0;
% electrical theta 120°-180°
elseif (2*pi/3 <= THETA) && (THETA < pi)
    H1 = 1;
    H2 = 1;
    H3 = 0;

% electrical theta 180°-240°
elseif (pi <= THETA) && (THETA < 4*pi/3)
    H1 = 0;
    H2 = 1;
    H3 = 0;

% electrical theta 240°-300°
elseif (4*pi/3 <= THETA) && (THETA < 5*pi/3)
    H1 = 0;
    H2 = 1;
    H3 = 1;

% electrical theta 300°-360°
elseif (5*pi/3 <= THETA) && (THETA < 2*pi)
    H1 = 0;
    H2 = 0;
    H3 = 1;

% something went wrong
else
    H1 = 0;
    H2 = 0;
    H3 = 0;
end

if CCW ~= 1
    if (H1 == 1) && (H3 == 1)
       S3 = 0; S2 = 0; S4 = 0; S5 = 0; S6 = 0;
       S1 = 1;
    elseif (H1 == 1) && (H2 ~= 1 && H3 ~= 1)
       S1 = 0; S4 = 0; S3 = 0; S5 = 0; S6 = 0;
       S2 = 1;
    elseif (H1 == 1) && (H2 == 1)
       S1 = 0; S2 = 0; S5 = 0; S4 = 0; S6 = 0;
       S3 = 1;
    elseif (H2 == 1) && (H1 ~= 1 && H3 ~= 1)
       S1 = 0; S2 = 0; S3 = 0; S6 = 0; S5 = 0;
       S4 = 1;
    elseif (H2 == 1) && (H3 == 1)
       S2 = 0; S3 = 0; S4 = 0; S1 = 0; S6 = 0;
       S5 = 1;
    elseif (H3 == 1) && (H1 ~= 1 && H2 ~= 1)
       S1 = 0; S3 = 0; S4 = 0; S5 = 0; S2 = 0;
       S6 = 1;
    else
       S1 = 0; S2 = 0; S3 = 0; S4 = 0; S5 = 0; S6 = 0; 
    end
else
    if (H1 == 1) && (H3 == 1)
       S3 = 0; S2 = 0; S1 = 0; S5 = 0; S6 = 0;
       S4 = 1;
    elseif (H1 == 1) && (H2 ~= 1 && H3 ~= 1)
       S1 = 0; S4 = 0; S3 = 0; S2 = 0; S6 = 0;
       S5 = 1;
    elseif (H1 == 1) && (H2 == 1)
       S1 = 0; S2 = 0; S5 = 0; S4 = 0; S3 = 0;
       S6 = 1;
    elseif (H2 == 1) && (H1 ~= 1 && H3 ~= 1)
       S4 = 0; S2 = 0; S3 = 0; S6 = 0; S5 = 0;
       S1 = 1;
    elseif (H2 == 1) && (H3 == 1)
       S5 = 0; S3 = 0; S4 = 0; S1 = 0; S6 = 0;
       S2 = 1;
    elseif (H3 == 1) && (H1 ~= 1 && H2 ~= 1)
       S1 = 0; S6 = 0; S4 = 0; S5 = 0; S2 = 0;
       S3 = 1;
    else
       S1 = 0; S2 = 0; S3 = 0; S4 = 0; S5 = 0; S6 = 0; 
    end
end

end

== matlab function 3DoFManipulatorWithBLDCM_SIMULATION/BLDC/Actuator Link0/Three Phase Inverter/MOTOR_SPEED_BLOCK1 ==
  data: U_U input; U_V input; U_W input; U_U_PWM output; PWM input; U_V_PWM output; U_W_PWM output
function [U_U_PWM, U_V_PWM, U_W_PWM] = PWM_SPEED_BLOCK(U_U, U_V, U_W, PWM)
%#codegen

%    This function was generated by the Symbolic Math Toolbox version 23.2.
%    20-Mar-2024 19:58:52

U_U_PWM = 0;
U_V_PWM = 0;
U_W_PWM = 0;

% Apply PWM scaling based on input and PWM signal
if U_U ~= 0 && PWM ~= 0
    U_U_PWM = U_U * PWM;
end
if U_V ~= 0 && PWM ~= 0
    U_V_PWM = U_V * PWM;
end
if U_W ~= 0 && PWM ~= 0
    U_W_PWM = U_W * PWM;
end

end
